simulink model "wind_DFIG"  (R2016a)
settings: Solver=ode23tb  StartTime=0.0  StopTime=50.0  RelTol=1e-4  AbsTol=1e-3
libraries: powerlib x8, powerlib_meascontrol x2, re_lib x1
settings Model: Creator=USER  LastModifiedBy=EBUKA
settings SolverCC: SolverResetMethod=Robust
settings GRTTargetCC: GeneratePreprocessorConditionals=Use local settings

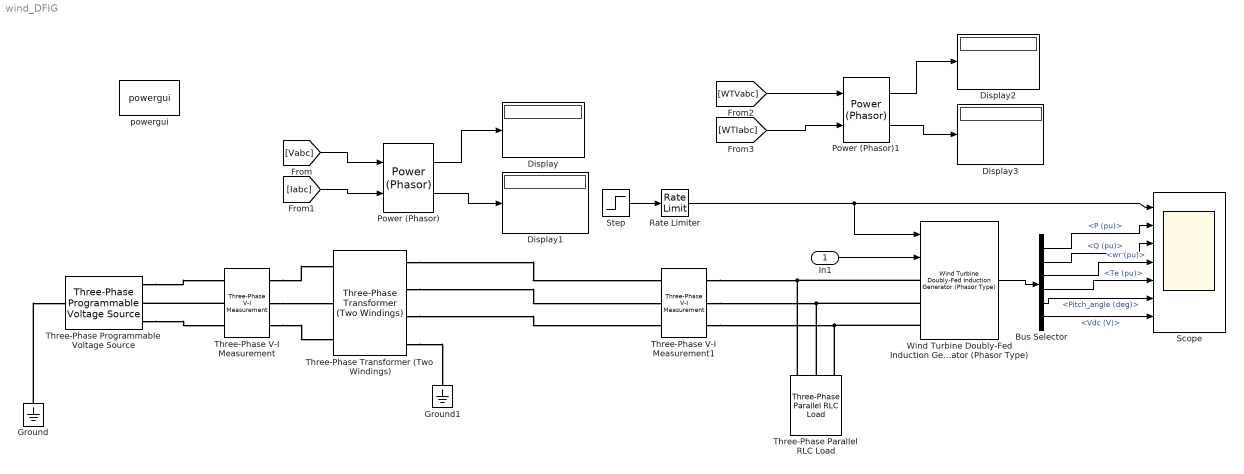
== system wind_DFIG ==
  In1 : Inport
  Bus Selector : BusSelector  OutputSignals=P (pu),Q (pu),wr (pu),Te (pu),Pitch_angle (deg),Vdc (V)
  Display{,1..3} (4 alike) : Display
  Ground : powerlib/Elements/Ground  LConnTagsString=a
  Ground1 : powerlib/Elements/Ground  LConnTagsString=a
  Power (Phasor) : powerlib_meascontrol/Measurements/Power (Phasor)
  Power (Phasor)1 : powerlib_meascontrol/Measurements/Power (Phasor)
  Rate Limiter : RateLimiter
  Scope : Scope  NumInputPorts=7
  Step : Step  Time=5  Before=8  After=14  SampleTime=0
  Three-Phase Parallel RLC Load : powerlib/Elements/Three-Phase Parallel RLC Load  LConnTagsString=A|B|C  Configuration=Y (grounded)  NominalVoltage=400  Vabc=[1e3 1e3 1e3]  Vabcp=[1e3 1e3 1e3]  NominalFrequency=50  UnbalancedPower=off  ActivePower=4e3  InductivePower=0  CapacitivePower=0  Pabc=[10e3 9e3 11e3]  QLabc=[100 90 110]  QCabc=[100 90 110]  Pabcp=[10e3 9e3 11e3]  QLabcp=[100 90 110]  QCabcp=[100 90 110]  Measurements=None  LoadType=constant Z
  Three-Phase Programmable Voltage Source : powerlib/Electrical Sources/Three-Phase Programmable Voltage Source  PositiveSequence="[25e3  0 50]"  VariationEntity=None  VariationType=Table of time-amplitude pairs  VariationTypeAlt=Step  VariationStep=0.5  VariationRate=10  VariationMagnitude=0.3  VariationFrequency=2  VariationTiming=[1 2]  VariationPhaseA=off  Amplitudes=[1 0.8 1.2 1.0]  TimeValues=[0 0.1 0.15 0.2]  HarmonicGeneration=off  HarmonicA=[3 0.2 -25 0]  HarmonicB=[2 0.15 35 2]  Timing="[0.05  3]"  BusType=swing  Pref=0  Qref=0  Qmin=-inf  Qmax=inf
  Three-Phase Transformer (Two Windings) : powerlib/Elements/Three-Phase Transformer (Two Windings)  Winding1Connection=Yg  Winding2Connection=Yn  CoreType=Three single-phase transformers  SetSaturation=off  Hysteresis=off  DataFile='hysteresis'  SetInitialFlux=off  Measurements=None  UNITS=pu  NominalPower=[ 4e6 , 50 ]  Winding1=[ 25e3 , 0.002 , 0.08 ]  Winding2=[ 400 , 0.002 , 0.08 ]  Rm=500  Lm=inf  L0=0.5  Saturation=[ 0,0 ; 0.0024,1.2 ; 1.0,1.52 ]  InitialFluxes=[ 0.8 , -0.8 , 0.7 ]  MoreParameters=off  BreakLoop=off  DataType=off  TransfoNumber=1
  Three-Phase V-I Measurement : powerlib/Measurements/Three-Phase V-I Measurement  VoltageMeasurement=phase-to-ground  SetLabelV=on  LabelV=Vabc  Vpu=off  VpuLL=off  CurrentMeasurement=yes  SetLabelI=on  LabelI=Iabc  Ipu=off  Pbase=100e6  Vbase=500e3  OutputType=Complex  PhasorSimulation=on  PSBequivalent=0
  Three-Phase V-I Measurement1 : powerlib/Measurements/Three-Phase V-I Measurement  VoltageMeasurement=phase-to-ground  SetLabelV=on  LabelV=WTVabc  Vpu=off  VpuLL=off  CurrentMeasurement=yes  SetLabelI=on  LabelI=WTIabc  Ipu=off  Pbase=100e6  Vbase=500e3  OutputType=Complex  PhasorSimulation=on  PSBequivalent=0
  Wind Turbine Doubly-Fed Induction Generator (Phasor Type) : re_lib/Wind Generation/Wind Turbine Doubly-Fed Induction Generator (Phasor Type)  ExternalTm=off  nom=[1e6 400 50]  sta=[ 0.00706 0.171]  rot=[ 0.005 0.156]  Lm=2.90  mec=[5.04 0.01 3]  init=[0.2 0 0 0 0 0]  speed_power=[0 0; 0.24 0.007; 0.36 0.024; 0.6 0.112; 0.96 0.46; 1.2 0.898; 1.5 0.898]  Pmec=1e6  speed_ABCD=[0.7 0.71 1.2 1.21]  power_C=0.73  wind_point_C=12  pitch_gain=500  pitch_max=45  pitch_rate=2  Pmax=0.5  Lchoke=[0.15 0.15/100]  init_inductor=[0 90]  Vdc_nom=1000  capacitor=10000e-6  ControlVQ=Voltage regulation  Vref=1.0  ExternalVref=off  Qref=1.0  ExternalQref=off  Iq_ref=0  ExternalIqref=off  Kpi_volt_reg=[1.25 300]  Xs=0.02  Kpi_Q=[0.05 5]  Kpi_power_reg=[1 100]  Kpi_dc_reg=[0.002 0.05]  Kpi_grid_side_cur_reg=[1 100]  Kpi_rotor_side_cur_reg=[0.3 8]  V_slew_rate=100  Q_slew_rate=100  power_slew_rate=1  current_slew_rate=200
  powergui : powerlib/powergui  Priority=1  SimulationMode=Phasor  SolverType=Tustin/Backward Euler (TBE)  SampleTime=50e-6  frequency=50  SPID=off  DisableSnubberDevices=off  DisableRonSwitches=off  DisableVfSwitches=off  SwTol=0  DisplayEquations=off  Interpol=off  ExternalGateDelay=off  methode=off  Ts=10  FunctionMessages=off  echomessages=off  HookPort=off  EnableUseOfTLC=off  x0status=blocks  frequencyindice=50  Pbase=100e6  ErrMax=1e-4  Iterations=50  UnitsV=kV  UnitsW=MW  buscounter=0  RestoreLinks=warning  ResistiveCurrentMeasurement=off  Frange=[0:2:500]  Ylog=off  Xlog=on  ShowGrid=off  save=off  variable=ZData  structure=0  ZoomFFT=off  StartTime=0.0  cycles=1  DisplayStyle=1  fundamental=60  FreqAxis=off  MaxFrequency=1000  frequencyindicesteady=1  RmsSteady=1  display=off
  wires:
  Step/1 -> Rate Limiter/1
  Wind Turbine Doubly-Fed Induction Generator (Phasor Type)/1 -> Bus Selector/1
  Bus Selector/5 -> Scope/6  "<Pitch_angle (deg)>"
  Bus Selector/4 -> Scope/5  "<Te (pu)>"
  Bus Selector/3 -> Scope/4  "<wr (pu)>"
  Bus Selector/2 -> Scope/3  "<Q (pu)>"
  Bus Selector/1 -> Scope/2  "<P (pu)>"
  [Vabc] -> Power (Phasor)/1
  [Iabc] -> Power (Phasor)/2
  Power (Phasor)/1 -> Display/1
  Power (Phasor)/2 -> Display1/1
  [WTVabc] -> Power (Phasor)1/1
  [WTIabc] -> Power (Phasor)1/2
  Power (Phasor)1/1 -> Display2/1
  Power (Phasor)1/2 -> Display3/1
  In1/1 -> Wind Turbine Doubly-Fed Induction Generator (Phasor Type)/2
  Bus Selector/6 -> Scope/7  "<Vdc (V)>"
  Rate Limiter/1 -> Wind Turbine Doubly-Fed Induction Generator (Phasor Type)/1, Scope/1
  connections:
  Three-Phase Parallel RLC Load/LConn1 -- Wind Turbine Doubly-Fed Induction Generator (Phasor Type)/LConn1 -- Three-Phase V-I Measurement1/RConn1
  Three-Phase Parallel RLC Load/LConn2 -- Wind Turbine Doubly-Fed Induction Generator (Phasor Type)/LConn2 -- Three-Phase V-I Measurement1/RConn2
  Three-Phase Parallel RLC Load/LConn3 -- Wind Turbine Doubly-Fed Induction Generator (Phasor Type)/LConn3 -- Three-Phase V-I Measurement1/RConn3
  Three-Phase V-I Measurement/LConn2 -- Three-Phase Programmable Voltage Source/RConn2
  Three-Phase V-I Measurement/RConn2 -- Three-Phase Transformer (Two Windings)/LConn2
  Three-Phase Transformer (Two Windings)/RConn4 -- Ground1/LConn1
  Three-Phase Programmable Voltage Source/RConn3 -- Three-Phase V-I Measurement/LConn3
  Three-Phase V-I Measurement/RConn3 -- Three-Phase Transformer (Two Windings)/LConn3
  Ground/LConn1 -- Three-Phase Programmable Voltage Source/LConn1
  Three-Phase Transformer (Two Windings)/RConn2 -- Three-Phase V-I Measurement1/LConn2
  Three-Phase Transformer (Two Windings)/RConn3 -- Three-Phase V-I Measurement1/LConn3
  Three-Phase Programmable Voltage Source/RConn1 -- Three-Phase V-I Measurement/LConn1
  Three-Phase Transformer (Two Windings)/RConn1 -- Three-Phase V-I Measurement1/LConn1
  Three-Phase V-I Measurement/RConn1 -- Three-Phase Transformer (Two Windings)/LConn1
